simulink model "PFC_dq_2019_temporelle_courant"  (R2023a)
settings: Solver=VariableStepAuto  StartTime=0.0  StopTime=temp_simu  RelTol=Te/20
undefined symbols (not defined in the file): C, Gamma_courant, i_de, K_courant, L, r, Rch, Te, Ud, Uq, w
settings Model: Creator=xshi  LastModifiedBy=dougl
settings SolverCC: AlgebraicLoopSolver=TrustRegion
settings DebuggingCC: UnconnectedInputMsg=warning  UnconnectedOutputMsg=warning  UnconnectedLineMsg=warning
settings ModelReferenceCC: EnableRefExpFcnMdlSchedulingChecks=on
settings SFSimCC: CustomCodeUndefinedFunction=UseInterfaceOnly

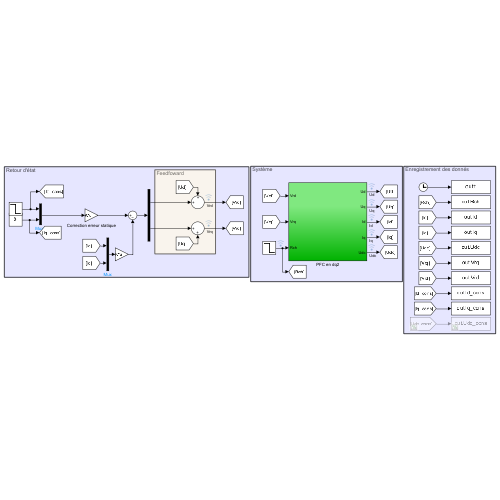
[thumbnail: Simulink's stored preview of the top-level diagram]
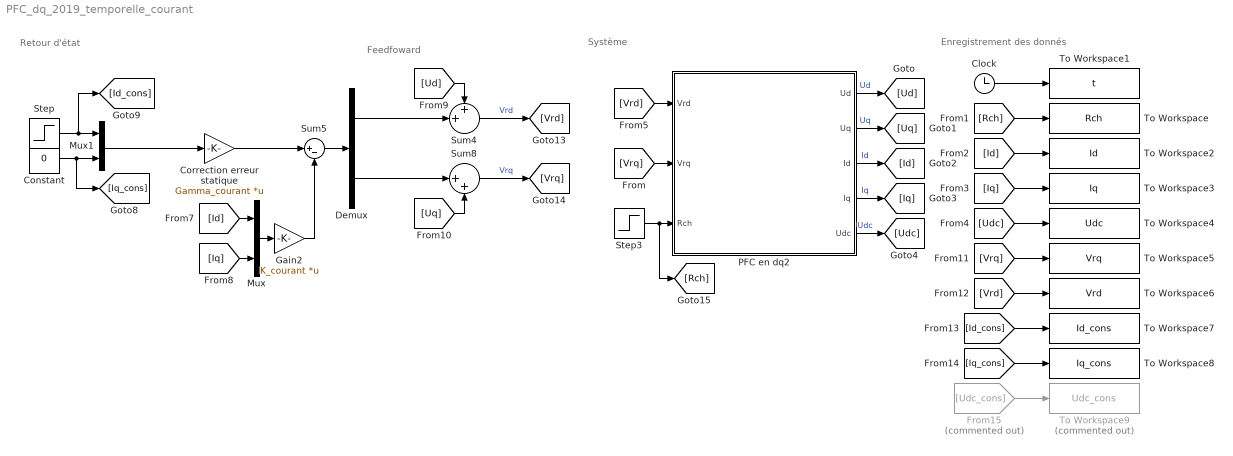
== system PFC_dq_2019_temporelle_courant ==
  note: Enregistrement des donnés
  note: Système
  note: Feedfoward
  note: Retour d'état
  Clock : Clock
  Constant : Constant  Value=0
  Correction erreur statique : Gain  Gain=Gamma_courant  Multiplication=Matrix(K*u)
  Demux : Demux  Outputs=2
  From15 : From  Commented=on  GotoTag=Udc_cons
  Gain2 : Gain  Gain=K_courant  Multiplication=Matrix(K*u)
  Mux : Mux  Inputs=2
  Mux1 : Mux  Inputs=2
  PFC en dq2 : Subsystem
  Step : Step  Before=i_de  After=i_de/2  SampleTime=0
  Step3 : Step  Time=3  Before=Rch  After=Rch/2  SampleTime=0
  Sum4 : Sum  Inputs=++|
  Sum5 : Sum  Inputs=|+-
  Sum8 : Sum  Inputs=|++
  To Workspace : ToWorkspace  VariableName=Rch  SampleTime=Te
  To Workspace1 : ToWorkspace  VariableName=t  SampleTime=Te
  To Workspace2 : ToWorkspace  VariableName=Id  SampleTime=Te
  To Workspace3 : ToWorkspace  VariableName=Iq  SampleTime=Te
  To Workspace4 : ToWorkspace  VariableName=Udc  SampleTime=Te
  To Workspace5 : ToWorkspace  VariableName=Vrq  SampleTime=Te
  To Workspace6 : ToWorkspace  VariableName=Vrd  SampleTime=Te
  To Workspace7 : ToWorkspace  VariableName=Id_cons  SampleTime=Te
  To Workspace8 : ToWorkspace  VariableName=Iq_cons  SampleTime=Te
  To Workspace9 : ToWorkspace  Commented=on  VariableName=Udc_cons  SampleTime=Te
  wires:
  Step3/1 -> PFC en dq2/3(Rch), [Rch]
  Sum8/1 -> [Vrq]  "Vrq"
  Sum4/1 -> [Vrd]  "Vrd"
  [Uq] -> Sum8/2
  Demux/2 -> Sum8/1
  Sum5/1 -> Demux/1
  [Id] -> Mux/1
  [Iq] -> Mux/2
  Mux/1 -> Gain2/1
  Correction erreur statique/1 -> Sum5/1
  Gain2/1 -> Sum5/2
  Demux/1 -> Sum4/2
  Mux1/1 -> Correction erreur statique/1
  [Ud] -> Sum4/1
  [Rch] -> To Workspace/1
  [Iq] -> To Workspace3/1
  [Vrd] -> To Workspace6/1
  [Vrq] -> To Workspace5/1
  [Udc] -> To Workspace4/1
  [Id_cons] -> To Workspace7/1
  [Iq_cons] -> To Workspace8/1
  From15/1 -> To Workspace9/1
  [Id] -> To Workspace2/1
  PFC en dq2/5(Udc) -> [Udc]  "Udc"
  PFC en dq2/2(Uq) -> [Uq]  "Uq"
  PFC en dq2/1(Ud) -> [Ud]  "Ud"
  PFC en dq2/3(Id) -> [Id]  "Id"
  PFC en dq2/4(Iq) -> [Iq]  "Iq"
  Clock/1 -> To Workspace1/1
  Constant/1 -> [Iq_cons], Mux1/2
  Step/1 -> [Id_cons], Mux1/1
  [Vrq] -> PFC en dq2/2(Vrq)
  [Vrd] -> PFC en dq2/1(Vrd)

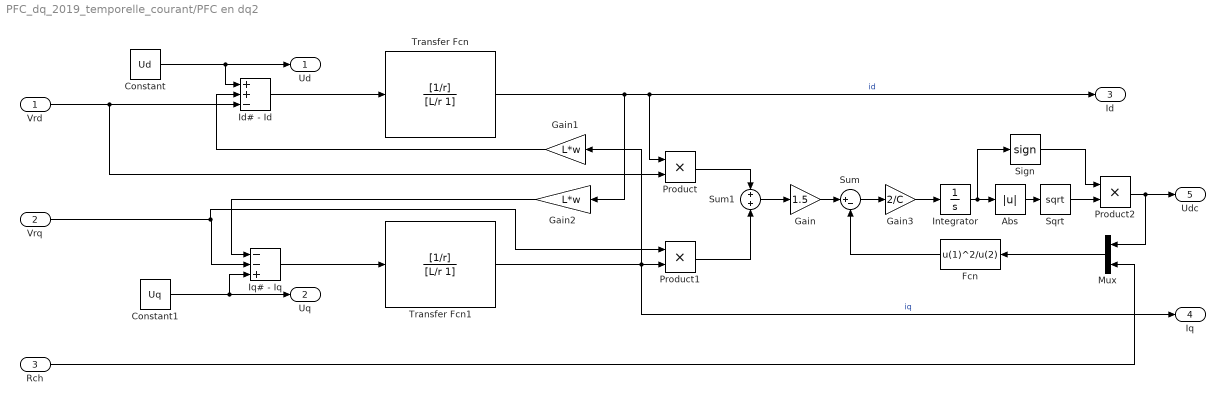
== system PFC_dq_2019_temporelle_courant/PFC en dq2 ==
  Vrd : Inport
  Vrq : Inport  Port=2
  Rch : Inport  Port=3
  Abs : Abs  SaturateOnIntegerOverflow=off
  Constant : Constant  Value=Ud
  Constant1 : Constant  Value=Uq
  Fcn : Fcn  Expr=u(1)^2/u(2)
  Gain : Gain  Gain=1.5
  Gain1 : Gain  Gain=L*w
  Gain2 : Gain  Gain=L*w
  Gain3 : Gain  Gain=2/C
  Id# - Id : Sum  Inputs=++-  InputSameDT=on  SaturateOnIntegerOverflow=on  OutDataTypeStr=Inherit: Same as first input
  Integrator : Integrator
  Iq# - Iq : Sum  Inputs=--+  InputSameDT=on  SaturateOnIntegerOverflow=on  OutDataTypeStr=Inherit: Same as first input
  Mux : Mux  Inputs=2
  Product : Product
  Product1 : Product
  Product2 : Product
  Sign : Signum
  Sqrt : Sqrt
  Sum : Sum  Inputs=|+-
  Sum1 : Sum
  Transfer Fcn : TransferFcn  Numerator=[1/r]  Denominator=[L/r 1]
  Transfer Fcn1 : TransferFcn  Numerator=[1/r]  Denominator=[L/r 1]
  Ud : Outport  VectorParamsAs1DForOutWhenUnconnected=off
  Uq : Outport  Port=2  VectorParamsAs1DForOutWhenUnconnected=off
  Id : Outport  Port=3  VectorParamsAs1DForOutWhenUnconnected=off
  Iq : Outport  Port=4  VectorParamsAs1DForOutWhenUnconnected=off
  Udc : Outport  Port=5  VectorParamsAs1DForOutWhenUnconnected=off
  wires:
  Sign/1 -> Product2/1
  Sqrt/1 -> Product2/2
  Abs/1 -> Sqrt/1
  Gain3/1 -> Integrator/1
  Mux/1 -> Fcn/1
  Sum/1 -> Gain3/1
  Integrator/1 -> Abs/1, Sign/1
  Fcn/1 -> Sum/2
  Gain/1 -> Sum/1
  Vrq/1 -> Product1/1, Iq# - Iq/2
  Rch/1 -> Mux/2
  Transfer Fcn1/1 -> Gain1/1, Product1/2, Iq/1  "iq"
  Gain1/1 -> Id# - Id/2
  Gain2/1 -> Iq# - Iq/1
  Id# - Id/1 -> Transfer Fcn/1
  Transfer Fcn/1 -> Product/1, Id/1, Gain2/1  "id"
  Vrd/1 -> Product/2, Id# - Id/3
  Constant/1 -> Ud/1, Id# - Id/1
  Iq# - Iq/1 -> Transfer Fcn1/1
  Constant1/1 -> Uq/1, Iq# - Iq/3
  Sum1/1 -> Gain/1
  Product/1 -> Sum1/1
  Product1/1 -> Sum1/2
  Product2/1 -> Mux/1, Udc/1
